simulink model "NOD"  (Simulink 6.3)
settings: Solver=FixedStepDiscrete  StartTime=0.0  StopTime=10.0  RelTol=1e-3
settings Model: LastModifiedBy=Umka  StrictBusMsg=None
settings DataIOCC: SignalLoggingName=sigsOut
settings DebuggingCC: SolverPrmCheckMsg=none
settings HardwareCC: TargetUnknown=on
settings STFCustomTargetCC: TargetFcnLib=ansi_tfl_tmw.mat  GenFloatMathFcnCalls=ANSI_C  ModelReferenceCompliant=off  SystemTargetFile=grt.tlc

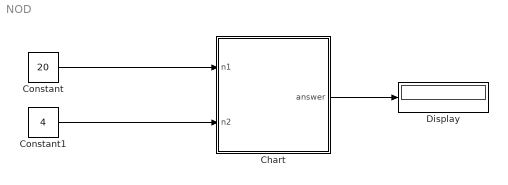
== system NOD ==
  Chart : Stateflow chart
  Constant : Constant  Value=20
  Constant1 : Constant  Value=4
  Display : Display
  wires:
  Constant/1 -> Chart/1(n1)
  Constant1/1 -> Chart/2(n2)
  Chart/1(answer) -> Display/1

== stateflow chart Chart ==
  state answer
  (default) -> (junction 4) : {nn1=n1,nn2=n2}
  (junction 4) -> (junction 5) [order 1] : [nn1<nn2]{nn2=nn2-nn1}
  (junction 5) -> (junction 4)
  (junction 4) -> answer [order 3] : {answer=nn1}
  (junction 6) -> (junction 4)
  (junction 4) -> (junction 6) [order 2] : [nn2<nn1]{nn1=nn1-nn2}
  data: n1 input double; n2 input double; answer output double; nn1 local double; nn2 local double
